simulink model "Simulink_template_R2019a"  (R2019a)
settings: Solver=ode1  StartTime=0.0  StopTime=1  FixedStep=0.0001  RelTol=1e-3
values from neighbouring files (symbols this model uses):
  inj_ang = [-90 -72 -54 -36 -18 0 18 36 54 72 90]    [table_data_save.m]    (also in test11_ForMakeData.m)
  inj_freq = [100 200 300 400 500]    [table_data_save.m]    (also in test11_ForMakeData.m)
  inj_volt = [1 5 10 15	20 25 30 35	40 45 50 55 60 65 70 75 80]    [table_data_save.m]    (also in test11_ForMakeData.m)
  table_data = zeros(11,17,5)    [table_data_save.m]
libraries: neural x55, simulink x5
(part 2 of 2)

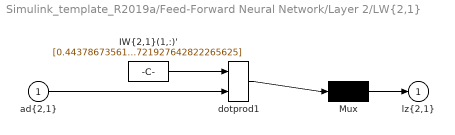
== system Simulink_template_R2019a/Feed-Forward Neural Network/Layer 2/LW{2,1} ==
  "ad{2,1}" : Inport  PortDimensions=50
      mask Display: e = 0.06;c1 = [120 230 180]/255;c2 = ([120 230 180]+0)/(256+128);c3 = ([120 230 180]+128)/(256+128);patch([0 1 1 0],[0 0 1 1],c1);patch([0 1 1 1-e 1-e 0+e],[0 0 1 1-e 0+e 0+e],c2);patch([0 0 1 1-e 0+e 0+e],[0 1 1 1-e 1-e 0+e],c3);plot([0 1 1 0 0],[0 0 1 1 0]);
  "IW{2,1}(1,:)'" : Constant  Value=[0.44378673561492865129451956818229518830776214599609375;-0.1053919464102655301207533966589835472404956817626953125;-0.7882791493778456004548615965177305042743682861328125;0.52511704606844433751433598445146344602108001708984375;-0.06678490339266361652814651961307390592992305755615234375;-0.70687533569330407434705421110265888273715972900390625;-1.255783505125525945089748347527347505092620849609375;0.07397619289665864628080527154452283866703510284423828125;0.111601339497780893683653857806348241865634918212890625;0.1701098105255012538084002926552784629166126251220703125;0.10816832609887494509592897884431295096874237060546875;-0.02893850365486012876647947678065975196659564971923828125;-1.0249754944344087181917757334304042160511016845703125;-0.0774492661348275268640151125509873963892459869384765625;0.0265206960658844574652004411063899169676005840301513671875;-0.197805703531938104067222639059764333069324493408203125;0.82300638620203525608332029150915332138538360595703125;0.0203749744933120376100266213370559853501617908477783203125;-0.82433238975160083583659798023290932178497314453125;0.006267778785131110190487202515896569821052253246307373046875;-0.1107499841702596909964739779752562753856182098388671875;-0.664681358723367310403773444704711437225341796875;0.2497333141776556519886298701749183237552642822265625;-0.35595763530203805569129826835705898702144622802734375;1.1343621976105147108881965323234908282756805419921875;0.047668587781283695836709313198298332281410694122314453125;0.0311190238149015620250370517396731884218752384185791015625;-0.9166014672967615073417846360825933516025543212890625;0.17931042422061482799477971639134921133518218994140625;-0.08467803669162000945735968571170815266668796539306640625;-0.7818871799200028949172747161355800926685333251953125;-2.089745048750019318362092235474847257137298583984375;0.1904098841118929408278148684985353611409664154052734375;1.51266984063729115206342612509615719318389892578125;-0.043358050798096438305240241106730536557734012603759765625;-1.4417515896001347197596942351083271205425262451171875;0.0297644995639530542119732814398957998491823673248291015625;-0.034672699984524803229479772426202544011175632476806640625;0.02292817166827813835094929117985884658992290496826171875;0.336151138802802063043628777450066991150379180908203125;1.4434887062302255156254204848664812743663787841796875;-0.0362931085957758636784120653828722424805164337158203125;0.044404643637456699123422509956071735359728336334228515625;0.39500857753399898353308117293636314570903778076171875;-0.388204871180458377377675560637726448476314544677734375;0.54699465423581850043177610132261179387569427490234375;-0.024415583573380465753910328885467606596648693084716796875;0.225606005805526865781729384252685122191905975341796875;-0.159449581686273267333575631710118614137172698974609375;0.323600000115878805306834919974789954721927642822265625]
      mask Display: e = 0.06;c1 = [120 150 230]/255;c2 = ([120 150 230]+0)/383;c3 = ([120 150 230]+128)/383;patch([0 1 1 0],[0 0 1 1],c1);patch([0 1 1 1-e 1-e 0+e],[0 0 1 1-e 0+e 0+e],c2);patch([0 0 1 1-e 0+e 0+e],[0 1 1 1-e 1-e 0+e],c3);plot([0 1 1 0 0],[0 0 1 1 0]);disp('weights');
  Mux : Mux  Inputs=1
      mask Display: e = 0.06;c1 = [120 150 230]/255;c2 = ([120 150 230]+0)/383;c3 = ([120 150 230]+128)/383;patch([0 1 1 0],[0 0 1 1],c1);patch([0 1 1 1-e 1-e 0+e],[0 0 1 1-e 0+e 0+e],c2);patch([0 0 1 1-e 0+e 0+e],[0 1 1 1-e 1-e 0+e],c3);plot([0 1 1 0 0],[0 0 1 1 0]);disp('Mux');
  dotprod1 : neural/Weight Functions/dotprod
  "lz{2,1}" : Outport
      mask Display: e = 0.06;c1 = [120 230 180]/255;c2 = ([120 230 180]+0)/(256+128);c3 = ([120 230 180]+128)/(256+128);patch([0 1 1 0],[0 0 1 1],c1);patch([0 1 1 1-e 1-e 0+e],[0 0 1 1-e 0+e 0+e],c2);patch([0 0 1 1-e 0+e 0+e],[0 1 1 1-e 1-e 0+e],c3);plot([0 1 1 0 0],[0 0 1 1 0]);
  wires:
  "IW{2,1}(1,:)'"/1 -> dotprod1/1
  "ad{2,1}"/1 -> dotprod1/2
  dotprod1/1 -> Mux/1
  Mux/1 -> "lz{2,1}"/1
